simulink model "PLFrameGenerator_var_est"  (R2022b)
settings: Solver=FixedStepAuto  StartTime=0.0  StopTime=19e-3  RelTol=1e-3
model workspace (MAT data in the model file):
  G = [1 0 0 0 0 0 1 0 1 0 0 0 ... (224 elements, 7x32)]
  HDRShortDUMMY : Simulink.LookupTable (value not decoded)
  PLSCLength = 90
  PilotMaxIdx = 1475
  PilotMinIdx = 1440
  Rsym = 10000000
  SNR : Simulink.Parameter (value not decoded)
  SOFLength = 26
  debugHeaderGain = 2
  mwTaskManagerKernelLatency = 0
  up_coef = 2
undefined symbols (not defined in the file or in its folder): Add, magnitude, Shift
libraries: simulink x15, hdlsllib x14, dsphdlfiltering2 x4, embmathops x4, dspsigops x3, commrandsrc3 x1, commfilt2 x1, dsphdlmathfun2 x1, commchan3 x1
(part 2 of 2)

== system PLFrameGenerator_var_est/Variance Estimator/Moving average ==
  enable : Inport
  dataIn : Inport  Port=2
  Add1 : Sum  Inputs=|+-  OutDataTypeStr=Inherit: Same as first input
  Add2 : Sum  Inputs=|++  OutDataTypeStr=Inherit: Same as first input
  Data Type Conversion : DataTypeConversion  OutDataTypeStr=double  SaturateOnIntegerOverflow=off  RndMeth=Floor
  Delay : Delay  DelayLength=2048  ShowEnablePort=on
      settings: InputPortMap=u0,e6
  Delay1 : Delay  DelayLength=1  ShowEnablePort=on
      settings: InputPortMap=u0,e6
  Delay{2,4..5,22} (4 alike) : Delay
  Delay3 : Delay  DelayLength=1  ShowEnablePort=on
      settings: InputPortMap=u0,e6
  Gain : Gain  Gain=1/2048  ParamDataTypeStr=fixdt(0,11,11)
  avgOut : Outport  InitialOutput=0
  wires:
  Delay3/1 -> avgOut/1
  Delay5/1 -> Delay1/2, Delay3/2
  Delay/1 -> Add1/2
  Add1/1 -> Delay22/1
  Delay22/1 -> Gain/1
  enable/1 -> Delay4/1, Delay/2
  Add2/1 -> Delay3/1, Delay1/1
  Delay1/1 -> Add2/2
  Delay2/1 -> Add2/1
  Data Type Conversion/1 -> Delay2/1
  Delay4/1 -> Delay5/1
  dataIn/1 -> Delay/1, Add1/1
  Gain/1 -> Data Type Conversion/1

== system PLFrameGenerator_var_est/FrameSynchronization/Correlator/MovingSum ==
  note: Delay by length of SoF sequence
  Scaled1 : Inport
  Scaled2 : Inport  Port=2
  ValidIn : Inport  Port=3
  Add : Sum  Inputs=|+-  OutDataTypeStr=Inherit: Same as first input
  Add1 : Sum  Inputs=|++  OutDataTypeStr=Inherit: Same as first input
  Add2 : Sum  Inputs=|+-  OutDataTypeStr=Inherit: Same as first input
  Add3 : Sum  Inputs=|++  OutDataTypeStr=Inherit: Same as first input
  Delay : Delay  DelayLength=26  ShowEnablePort=on
      settings: InputPortMap=u0,e6
  Delay1 : Delay  DelayLength=64  ShowEnablePort=on
      settings: InputPortMap=u0,e6
  Delay14 : Delay  DelayLength=1  ShowEnablePort=on
      settings: InputPortMap=u0,e6
  Delay2 : Delay  DelayLength=1  ShowEnablePort=on
      settings: InputPortMap=u0,e6
  E1 : Outport
  E2 : Outport  Port=2
  wires:
  Scaled1/1 -> Add/1, Delay/1
  Delay/1 -> Add/2
  Add/1 -> Add1/1
  Delay14/1 -> Add1/2
  Scaled2/1 -> Delay1/1, Add2/1
  Delay1/1 -> Add2/2
  ValidIn/1 -> Delay1/2, Delay/2, Delay14/2, Delay2/2
  Add2/1 -> Add3/1
  Delay2/1 -> Add3/2
  Add3/1 -> Delay2/1, E2/1
  Add1/1 -> E1/1, Delay14/1

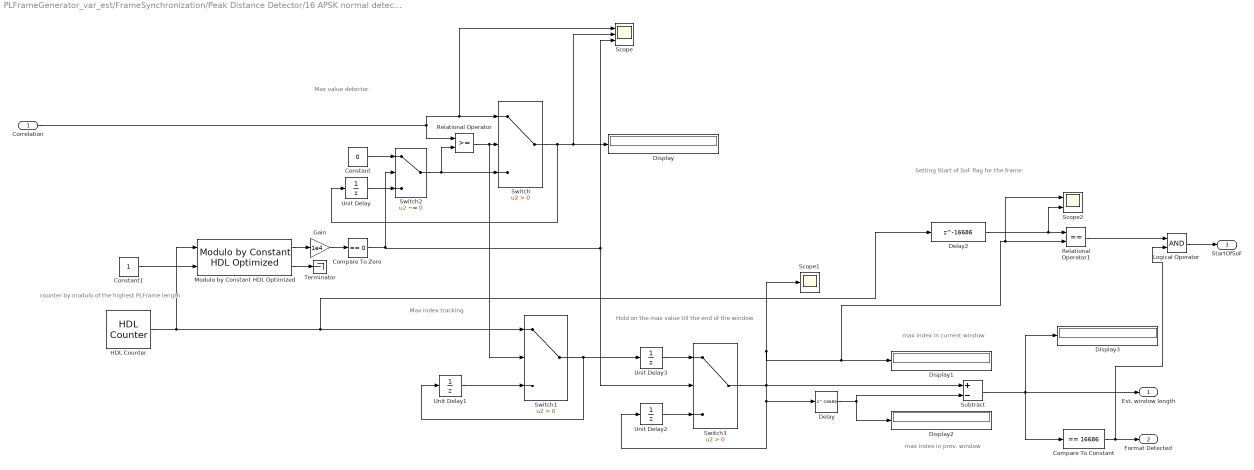
== system PLFrameGenerator_var_est/FrameSynchronization/Peak Distance Detector/16 APSK normal detector ==
  note: Max value detector
  note: Hold on the max value till the end of the window
  note: Max index tracking
  note: max index in current window
  note: max index in prev. window
  note: counter by modulo of the highest PLFrame length
  note: Setting Start of SoF flag for the frame
  Correlation : Inport
  Compare To Constant : simulink/Logic and Bit Operations/Compare To Constant  relop===  const=16686  OutDataTypeStr=boolean
  Compare To Zero : simulink/Logic and Bit Operations/Compare To Zero  relop===  OutDataTypeStr=boolean
  Constant : Constant  Value=0  SampleTime=-1
  Constant1 : Constant  OutDataTypeStr=boolean  SampleTime=-1
  Delay : Delay  DelayLength=16686
  Delay2 : Delay  DelayLength=16686
  Display{,1..3} (4 alike) : Display
      settings: Format=long_e
  Gain : Gain  Gain=1e4
  HDL Counter : hdlsllib/Sources/HDL Counter  CountType=Modulo  CountInit=0  CountStep=1  CountMax=2^32-1  CountFromType=Initial value  CountFrom=0  CountResetPort=off  CountLoadPort=off  CountEnbPort=off  CountDirPort=off  CountHitOutputPort=off  CountDataType=Unsigned  CountWordLen=32  CountFracLen=0  CountSampTime=-1
  Logical Operator : Logic  AllPortsSameDT=off  OutDataTypeStr=boolean
  Modulo by Constant HDL Optimized : embmathops/Modulo by Constant HDL Optimized  Denominator=16686  SimulateUsing=Code generation
      settings: LibrarySourceBlock=|
      | embeddedMatrixLib/Math Operations/Modulo by Constant
      | HDL Optimized
  Relational Operator : RelationalOperator  OutDataTypeStr=boolean  RndMeth=Simplest  InputSameDT=off
  Relational Operator1 : RelationalOperator  Operator===  OutDataTypeStr=boolean  RndMeth=Simplest  InputSameDT=off
  Scope : Scope  NumInputPorts=3
  Scope1 : Scope
  Scope2 : Scope  NumInputPorts=2
  Subtract : Sum  Inputs=+-
  Switch : Switch  Criteria=u2 > Threshold  SaturateOnIntegerOverflow=off  InputSameDT=off
  Switch1 : Switch  Criteria=u2 > Threshold  SaturateOnIntegerOverflow=off  InputSameDT=off
  Switch2 : Switch  Criteria=u2 ~= 0  SaturateOnIntegerOverflow=off  InputSameDT=off
  Switch3 : Switch  Criteria=u2 > Threshold  SaturateOnIntegerOverflow=off  InputSameDT=off
  Terminator : Terminator
  Unit Delay{,1..3} (4 alike) : UnitDelay  SampleTime=-1  HasFrameUpgradeWarning=on
  Est. window length : Outport
  Format Detected : Outport  Port=2
  StartOfSoF : Outport  Port=3
  wires:
  Unit Delay/1 -> Switch2/3
  Unit Delay2/1 -> Switch3/3
  Correlation/1 -> Scope/1, Switch/1, Relational Operator/1
  Compare To Zero/1 -> Switch3/2, Scope/3, Switch2/2
  Switch/1 -> Unit Delay/1, Display/1, Scope/2
  Modulo by Constant HDL Optimized/1 -> Gain/1
  Unit Delay1/1 -> Switch1/3
  Relational Operator/1 -> Switch1/2, Switch/2
  Switch2/1 -> Switch/3, Relational Operator/2
  Delay/1 -> Subtract/2, Display2/1
  Constant1/1 -> Modulo by Constant HDL Optimized/2
  Subtract/1 -> Compare To Constant/1, Display3/1, Est. window length/1
  Constant/1 -> Switch2/1
  Switch1/1 -> Unit Delay1/1, Unit Delay3/1
  Gain/1 -> Compare To Zero/1
  Modulo by Constant HDL Optimized/2 -> Terminator/1
  Unit Delay3/1 -> Switch3/1
  HDL Counter/1 -> Modulo by Constant HDL Optimized/1, Delay2/1, Switch1/1
  Relational Operator1/1 -> Logical Operator/1
  Compare To Constant/1 -> Logical Operator/2, Format Detected/1
  Delay2/1 -> Scope2/2, Relational Operator1/1
  Switch3/1 -> Subtract/1, Scope1/1, Relational Operator1/2, Scope2/1, Display1/1, Unit Delay2/1, Delay/1
  Logical Operator/1 -> StartOfSoF/1

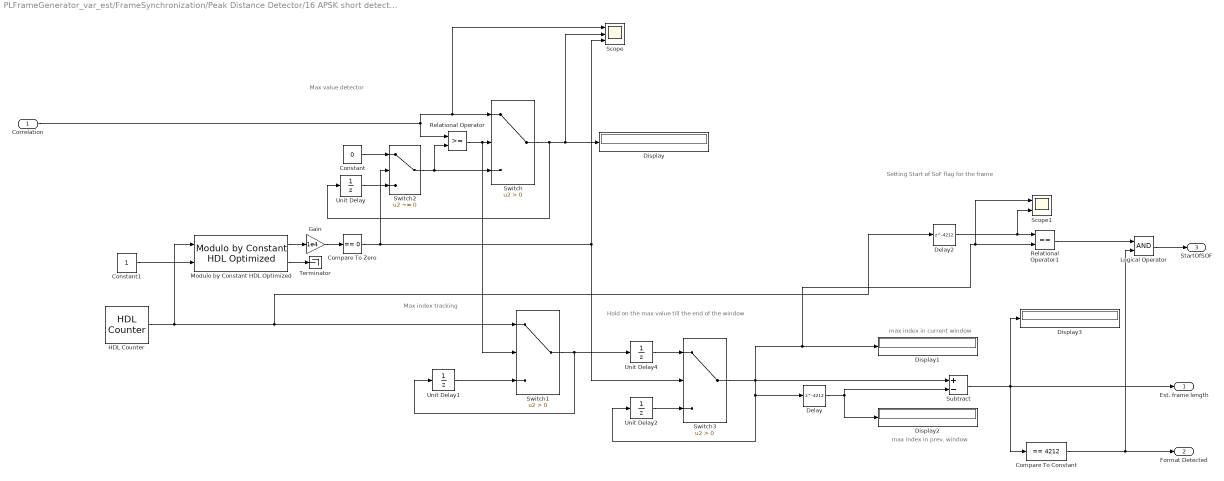
== system PLFrameGenerator_var_est/FrameSynchronization/Peak Distance Detector/16 APSK short detector ==
  note: Setting Start of SoF flag for the frame
  note: Max value detector
  note: Hold on the max value till the end of the window
  note: Max index tracking
  note: max index in current window
  note: max index in prev. window
  Correlation : Inport
  Compare To Constant : simulink/Logic and Bit Operations/Compare To Constant  relop===  const=4212  OutDataTypeStr=boolean
  Compare To Zero : simulink/Logic and Bit Operations/Compare To Zero  relop===  OutDataTypeStr=boolean
  Constant : Constant  Value=0  SampleTime=-1
  Constant1 : Constant  OutDataTypeStr=boolean  SampleTime=-1
  Delay : Delay  DelayLength=4212
  Delay2 : Delay  DelayLength=4212
  Display{,1..3} (4 alike) : Display
      settings: Format=long_e
  Gain : Gain  Gain=1e4
  HDL Counter : hdlsllib/Sources/HDL Counter  CountType=Modulo  CountInit=0  CountStep=1  CountMax=2^32-1  CountFromType=Initial value  CountFrom=0  CountResetPort=off  CountLoadPort=off  CountEnbPort=off  CountDirPort=off  CountHitOutputPort=off  CountDataType=Unsigned  CountWordLen=32  CountFracLen=0  CountSampTime=-1
  Logical Operator : Logic  AllPortsSameDT=off  OutDataTypeStr=boolean
  Modulo by Constant HDL Optimized : embmathops/Modulo by Constant HDL Optimized  Denominator=4212  SimulateUsing=Code generation
      settings: LibrarySourceBlock=|
      | embeddedMatrixLib/Math Operations/Modulo by Constant
      | HDL Optimized
  Relational Operator : RelationalOperator  OutDataTypeStr=boolean  RndMeth=Simplest  InputSameDT=off
  Relational Operator1 : RelationalOperator  Operator===  OutDataTypeStr=boolean  RndMeth=Simplest  InputSameDT=off
  Scope : Scope  NumInputPorts=3
  Scope1 : Scope  NumInputPorts=2
  Subtract : Sum  Inputs=+-
  Switch : Switch  Criteria=u2 > Threshold  SaturateOnIntegerOverflow=off  InputSameDT=off
  Switch1 : Switch  Criteria=u2 > Threshold  SaturateOnIntegerOverflow=off  InputSameDT=off
  Switch2 : Switch  Criteria=u2 ~= 0  SaturateOnIntegerOverflow=off  InputSameDT=off
  Switch3 : Switch  Criteria=u2 > Threshold  SaturateOnIntegerOverflow=off  InputSameDT=off
  Terminator : Terminator
  Unit Delay{,1..2,4} (4 alike) : UnitDelay  SampleTime=-1  HasFrameUpgradeWarning=on
  Est. frame length : Outport
  Format Detected : Outport  Port=2
  StartOfSOF : Outport  Port=3
  wires:
  Unit Delay/1 -> Switch2/3
  Unit Delay2/1 -> Switch3/3
  Correlation/1 -> Scope/1, Switch/1, Relational Operator/1
  Switch3/1 -> Subtract/1, Relational Operator1/2, Scope1/1, Display1/1, Unit Delay2/1, Delay/1
  Switch/1 -> Unit Delay/1, Display/1, Scope/2
  Modulo by Constant HDL Optimized/1 -> Gain/1
  Unit Delay1/1 -> Switch1/3
  Relational Operator/1 -> Switch1/2, Switch/2
  Switch2/1 -> Switch/3, Relational Operator/2
  Delay/1 -> Subtract/2, Display2/1
  Constant1/1 -> Modulo by Constant HDL Optimized/2
  Subtract/1 -> Compare To Constant/1, Display3/1, Est. frame length/1
  Constant/1 -> Switch2/1
  Switch1/1 -> Unit Delay1/1, Unit Delay4/1
  Gain/1 -> Compare To Zero/1
  HDL Counter/1 -> Modulo by Constant HDL Optimized/1, Delay2/1, Switch1/1
  Modulo by Constant HDL Optimized/2 -> Terminator/1
  Compare To Constant/1 -> Format Detected/1, Logical Operator/2
  Compare To Zero/1 -> Scope/3, Switch3/2, Switch2/2
  Unit Delay4/1 -> Switch3/1
  Delay2/1 -> Scope1/2, Relational Operator1/1
  Relational Operator1/1 -> Logical Operator/1
  Logical Operator/1 -> StartOfSOF/1

== system PLFrameGenerator_var_est/FrameSynchronization/Peak Distance Detector/Decision Block ==
  note: start of SOF here
  note: 8 16APSK short Valid (1 input)
      | 4 16 APSK normal Valid (2 input)
      | 2 QPSK short Valid (3 input)
      | 1 QPSK normal Valid (4 input)
      | 0 frame sync not achieved yet
  16APSK short Valid : Inport
  16APSK short start of SOF : Inport  Port=2
  16APSK normal Valid : Inport  Port=3
  16APSK normal start of SOF : Inport  Port=4
  QPSK short Valid : Inport  Port=5
  QPSK short start of SOF : Inport  Port=6
  QPSK normal Valid : Inport  Port=7
  QPSK normal start of SOF : Inport  Port=8
  Constant : Constant  Value=0  OutDataTypeStr=boolean  SampleTime=-1
  Decision : Subsystem
  Delay1 : Delay  DelayLength=37
  Delay4 : Delay  DelayLength=SOFLength
  Header Valid Indicator : Subsystem
  Scope : Scope
  Start of SOF Switch : MultiPortSwitch  DataPortOrder=Specify indices  Inputs=5  DataPortIndices={8, 4, 2, 1, 0}  SaturateOnIntegerOverflow=off  InputSameDT=off
  EndOfSOD : Outport
  FrameSync success : Outport  Port=2
  HeaderValid : Outport  Port=3
  wires:
  16APSK short start of SOF/1 -> Start of SOF Switch/2
  16APSK normal start of SOF/1 -> Start of SOF Switch/3
  QPSK short start of SOF/1 -> Start of SOF Switch/4
  QPSK normal start of SOF/1 -> Start of SOF Switch/5
  16APSK short Valid/1 -> Decision/1(16APSK short Valid)
  16APSK normal Valid/1 -> Decision/2(16APSK normal Valid)
  QPSK short Valid/1 -> Decision/3(QPSK short Valid)
  QPSK normal Valid/1 -> Decision/4(QPSK normal Valid)
  Delay1/1 -> Delay4/1, Header Valid Indicator/1(Start of SOF)
  Delay4/1 -> EndOfSOD/1
  Header Valid Indicator/1(PLFrameHDRValid) -> HeaderValid/1
  Start of SOF Switch/1 -> Scope/1, Delay1/1
  Decision/1(FrameSync success) -> FrameSync success/1
  Decision/2(Decision Output) -> Start of SOF Switch/1
  Constant/1 -> Start of SOF Switch/6

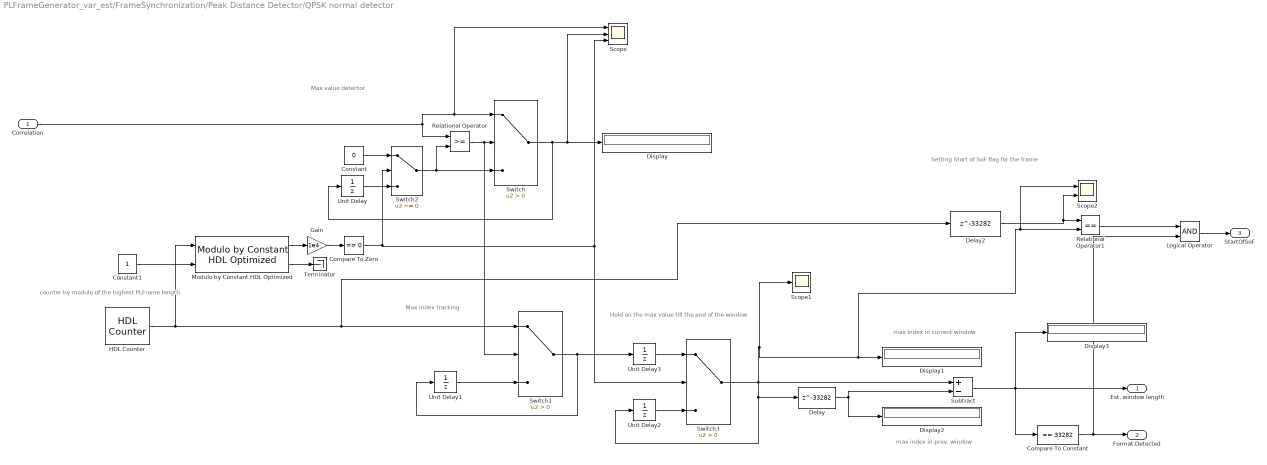
== system PLFrameGenerator_var_est/FrameSynchronization/Peak Distance Detector/QPSK normal detector ==
  note: Max value detector
  note: Hold on the max value till the end of the window
  note: Max index tracking
  note: max index in current window
  note: max index in prev. window
  note: counter by modulo of the highest PLFrame length
  note: Setting Start of SoF flag for the frame
  Correlation : Inport
  Compare To Constant : simulink/Logic and Bit Operations/Compare To Constant  relop===  const=33282  OutDataTypeStr=boolean
  Compare To Zero : simulink/Logic and Bit Operations/Compare To Zero  relop===  OutDataTypeStr=boolean
  Constant : Constant  Value=0  SampleTime=-1
  Constant1 : Constant  OutDataTypeStr=boolean  SampleTime=-1
  Delay : Delay  DelayLength=33282
  Delay2 : Delay  DelayLength=33282
  Display{,1..3} (4 alike) : Display
      settings: Format=long_e
  Gain : Gain  Gain=1e4
  HDL Counter : hdlsllib/Sources/HDL Counter  CountType=Modulo  CountInit=0  CountStep=1  CountMax=2^32-1  CountFromType=Initial value  CountFrom=0  CountResetPort=off  CountLoadPort=off  CountEnbPort=off  CountDirPort=off  CountHitOutputPort=off  CountDataType=Unsigned  CountWordLen=32  CountFracLen=0  CountSampTime=-1
  Logical Operator : Logic  AllPortsSameDT=off  OutDataTypeStr=boolean
  Modulo by Constant HDL Optimized : embmathops/Modulo by Constant HDL Optimized  Denominator=33282  SimulateUsing=Code generation
      settings: LibrarySourceBlock=|
      | embeddedMatrixLib/Math Operations/Modulo by Constant
      | HDL Optimized
  Relational Operator : RelationalOperator  OutDataTypeStr=boolean  RndMeth=Simplest  InputSameDT=off
  Relational Operator1 : RelationalOperator  Operator===  OutDataTypeStr=boolean  RndMeth=Simplest  InputSameDT=off
  Scope : Scope  NumInputPorts=3
  Scope1 : Scope
  Scope2 : Scope  NumInputPorts=2
  Subtract : Sum  Inputs=+-
  Switch : Switch  Criteria=u2 > Threshold  SaturateOnIntegerOverflow=off  InputSameDT=off
  Switch1 : Switch  Criteria=u2 > Threshold  SaturateOnIntegerOverflow=off  InputSameDT=off
  Switch2 : Switch  Criteria=u2 ~= 0  SaturateOnIntegerOverflow=off  InputSameDT=off
  Switch3 : Switch  Criteria=u2 > Threshold  SaturateOnIntegerOverflow=off  InputSameDT=off
  Terminator : Terminator
  Unit Delay{,1..3} (4 alike) : UnitDelay  SampleTime=-1  HasFrameUpgradeWarning=on
  Est. window length : Outport
  Format Detected : Outport  Port=2
  StartOfSoF : Outport  Port=3
  wires:
  Unit Delay/1 -> Switch2/3
  Unit Delay2/1 -> Switch3/3
  Correlation/1 -> Scope/1, Switch/1, Relational Operator/1
  Compare To Zero/1 -> Switch3/2, Scope/3, Switch2/2
  Switch/1 -> Unit Delay/1, Display/1, Scope/2
  Modulo by Constant HDL Optimized/1 -> Gain/1
  Unit Delay1/1 -> Switch1/3
  Relational Operator/1 -> Switch1/2, Switch/2
  Switch2/1 -> Switch/3, Relational Operator/2
  Delay/1 -> Subtract/2, Display2/1
  Constant1/1 -> Modulo by Constant HDL Optimized/2
  Subtract/1 -> Compare To Constant/1, Display3/1, Est. window length/1
  Constant/1 -> Switch2/1
  Switch1/1 -> Unit Delay1/1, Unit Delay3/1
  Gain/1 -> Compare To Zero/1
  Modulo by Constant HDL Optimized/2 -> Terminator/1
  Unit Delay3/1 -> Switch3/1
  Logical Operator/1 -> StartOfSoF/1
  Delay2/1 -> Scope2/2, Relational Operator1/1
  Relational Operator1/1 -> Logical Operator/1
  Switch3/1 -> Subtract/1, Scope1/1, Relational Operator1/2, Scope2/1, Display1/1, Unit Delay2/1, Delay/1
  HDL Counter/1 -> Modulo by Constant HDL Optimized/1, Delay2/1, Switch1/1
  Compare To Constant/1 -> Format Detected/1, Logical Operator/2

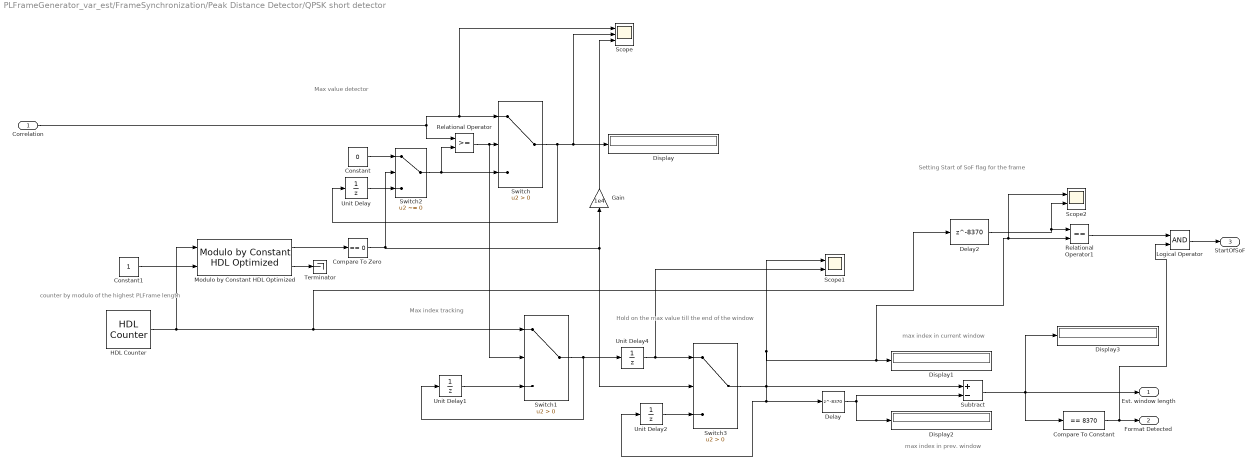
== system PLFrameGenerator_var_est/FrameSynchronization/Peak Distance Detector/QPSK short detector ==
  note: Max value detector
  note: Hold on the max value till the end of the window
  note: Max index tracking
  note: max index in current window
  note: max index in prev. window
  note: counter by modulo of the highest PLFrame length
  note: Setting Start of SoF flag for the frame
  Correlation : Inport
  Compare To Constant : simulink/Logic and Bit Operations/Compare To Constant  relop===  const=8370  OutDataTypeStr=boolean
  Compare To Zero : simulink/Logic and Bit Operations/Compare To Zero  relop===  OutDataTypeStr=boolean
  Constant : Constant  Value=0  SampleTime=-1
  Constant1 : Constant  OutDataTypeStr=boolean  SampleTime=-1
  Delay : Delay  DelayLength=8370
  Delay2 : Delay  DelayLength=8370
  Display{,1..3} (4 alike) : Display
      settings: Format=long_e
  Gain : Gain  Gain=1e4
  HDL Counter : hdlsllib/Sources/HDL Counter  CountType=Modulo  CountInit=0  CountStep=1  CountMax=2^32-1  CountFromType=Initial value  CountFrom=0  CountResetPort=off  CountLoadPort=off  CountEnbPort=off  CountDirPort=off  CountHitOutputPort=off  CountDataType=Unsigned  CountWordLen=32  CountFracLen=0  CountSampTime=-1
  Logical Operator : Logic  AllPortsSameDT=off  OutDataTypeStr=boolean
  Modulo by Constant HDL Optimized : embmathops/Modulo by Constant HDL Optimized  Denominator=8370  SimulateUsing=Code generation
      settings: LibrarySourceBlock=|
      | embeddedMatrixLib/Math Operations/Modulo by Constant
      | HDL Optimized
  Relational Operator : RelationalOperator  OutDataTypeStr=boolean  RndMeth=Simplest  InputSameDT=off
  Relational Operator1 : RelationalOperator  Operator===  OutDataTypeStr=boolean  RndMeth=Simplest  InputSameDT=off
  Scope : Scope  NumInputPorts=3
  Scope1 : Scope  NumInputPorts=2
  Scope2 : Scope  NumInputPorts=2
  Subtract : Sum  Inputs=+-
  Switch : Switch  Criteria=u2 > Threshold  SaturateOnIntegerOverflow=off  InputSameDT=off
  Switch1 : Switch  Criteria=u2 > Threshold  SaturateOnIntegerOverflow=off  InputSameDT=off
  Switch2 : Switch  Criteria=u2 ~= 0  SaturateOnIntegerOverflow=off  InputSameDT=off
  Switch3 : Switch  Criteria=u2 > Threshold  SaturateOnIntegerOverflow=off  InputSameDT=off
  Terminator : Terminator
  Unit Delay{,1..2,4} (4 alike) : UnitDelay  SampleTime=-1  HasFrameUpgradeWarning=on
  Est. window length : Outport
  Format Detected : Outport  Port=2
  StartOfSoF : Outport  Port=3
  wires:
  Unit Delay/1 -> Switch2/3
  Unit Delay2/1 -> Switch3/3
  Correlation/1 -> Scope/1, Switch/1, Relational Operator/1
  Switch/1 -> Unit Delay/1, Display/1, Scope/2
  Unit Delay1/1 -> Switch1/3
  Relational Operator/1 -> Switch1/2, Switch/2
  Switch2/1 -> Switch/3, Relational Operator/2
  Delay/1 -> Subtract/2, Display2/1
  Constant1/1 -> Modulo by Constant HDL Optimized/2
  Subtract/1 -> Compare To Constant/1, Display3/1, Est. window length/1
  Constant/1 -> Switch2/1
  Modulo by Constant HDL Optimized/1 -> Compare To Zero/1
  Modulo by Constant HDL Optimized/2 -> Terminator/1
  Gain/1 -> Scope/3
  Switch1/1 -> Unit Delay4/1, Unit Delay1/1
  Compare To Zero/1 -> Switch3/2, Gain/1, Switch2/2
  Unit Delay4/1 -> Scope1/2, Switch3/1
  Logical Operator/1 -> StartOfSoF/1
  Delay2/1 -> Scope2/2, Relational Operator1/1
  Relational Operator1/1 -> Logical Operator/1
  Switch3/1 -> Subtract/1, Scope1/1, Relational Operator1/2, Scope2/1, Display1/1, Unit Delay2/1, Delay/1
  HDL Counter/1 -> Modulo by Constant HDL Optimized/1, Delay2/1, Switch1/1
  Compare To Constant/1 -> Logical Operator/2, Format Detected/1

== system PLFrameGenerator_var_est/FrameSynchronization/Peak Distance Detector/Decision Block/Decision ==
  16APSK short Valid : Inport
  16APSK normal Valid : Inport  Port=2
  QPSK short Valid : Inport  Port=3
  QPSK normal Valid : Inport  Port=4
  Bit Concat : hdlsllib/Logic and Bit Operations/Bit Concat  numInputs=2
  Bit Concat1 : hdlsllib/Logic and Bit Operations/Bit Concat  numInputs=2
  Bit Concat2 : hdlsllib/Logic and Bit Operations/Bit Concat  numInputs=2
  Display{,1..6} (7 alike) : Display
  Logical Operator : Logic  Operator=OR  Inputs=4  AllPortsSameDT=off  OutDataTypeStr=boolean
  FrameSync success : Outport
  Decision Output : Outport  Port=2
  wires:
  16APSK short Valid/1 -> Logical Operator/1, Display3/1, Bit Concat/1
  16APSK normal Valid/1 -> Logical Operator/2, Display4/1, Bit Concat/2
  QPSK short Valid/1 -> Logical Operator/3, Display6/1, Bit Concat1/1
  QPSK normal Valid/1 -> Logical Operator/4, Bit Concat1/2, Display5/1
  Bit Concat/1 -> Bit Concat2/1, Display1/1
  Bit Concat1/1 -> Display2/1, Bit Concat2/2
  Bit Concat2/1 -> Decision Output/1, Display/1
  Logical Operator/1 -> FrameSync success/1

== system PLFrameGenerator_var_est/FrameSynchronization/Peak Distance Detector/Decision Block/Header Valid Indicator ==
  Start of SOF : Inport
  Compare To Zero : simulink/Logic and Bit Operations/Compare To Zero  relop=~=  OutDataTypeStr=boolean
  HDL Counter1 : hdlsllib/Sources/HDL Counter  CountType=Count limited  CountInit=0  CountStep=1  CountMax=89  CountFromType=Initial value  CountFrom=0  CountResetPort=on  CountLoadPort=off  CountEnbPort=off  CountDirPort=off  CountHitOutputPort=off  CountDataType=Unsigned  CountWordLen=8  CountFracLen=0  CountSampTime=1
  IsZero : simulink/Logic and Bit Operations/Compare To Zero  relop===  OutDataTypeStr=boolean
      settings: LibrarySourceBlock=|
      | simulink/Quick Insert/Logic and Bit
      | Operations/IsZero
  Logical Operator : Logic  AllPortsSameDT=off  OutDataTypeStr=boolean
  Logical Operator1 : Logic  AllPortsSameDT=off  OutDataTypeStr=boolean
  Logical Operator2 : Logic  Operator=OR  AllPortsSameDT=off  OutDataTypeStr=boolean
  NOT : Logic  Operator=NOT  IconShape=distinctive  AllPortsSameDT=off  OutDataTypeStr=boolean
  NOT1 : Logic  Operator=NOT  IconShape=distinctive  AllPortsSameDT=off  OutDataTypeStr=boolean
  Unit Delay : UnitDelay  SampleTime=-1  HasFrameUpgradeWarning=on
  PLFrameHDRValid : Outport
  wires:
  HDL Counter1/1 -> IsZero/1, Compare To Zero/1
  NOT/1 -> Logical Operator/2
  Compare To Zero/1 -> Logical Operator2/2
  NOT1/1 -> Logical Operator1/1
  Logical Operator/1 -> NOT1/1, HDL Counter1/1
  Logical Operator1/1 -> Logical Operator2/1
  IsZero/1 -> Logical Operator1/2, Logical Operator/1
  Start of SOF/1 -> Unit Delay/1
  Logical Operator2/1 -> PLFrameHDRValid/1
  Unit Delay/1 -> NOT/1
